simulink model "chap04_01_03_mdl"  (R2013b)
settings: Solver=ode45  StartTime=0.0  StopTime=10.0  RelTol=1e-3
settings Model: Creator=Administrator  LastModifiedBy=sunzx.fnst

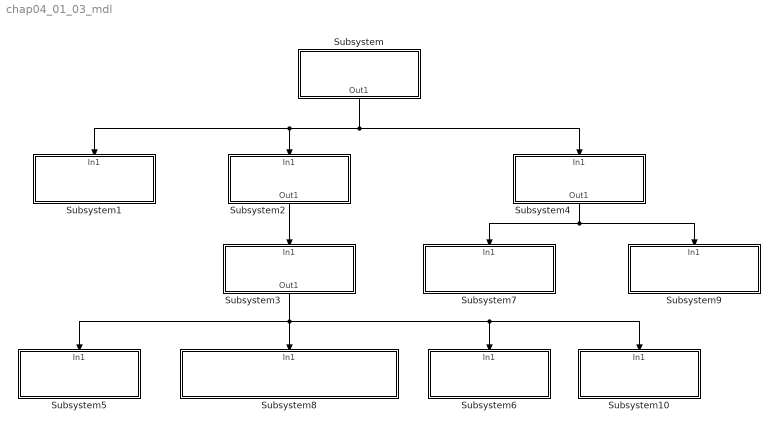
== system chap04_01_03_mdl ==
  Subsystem : Subsystem
      mask Display: disp('Subsystem');
  Subsystem1 : Subsystem
      mask Display: disp('Virtrual Subsystem');
  Subsystem10 : Subsystem
      mask Display: disp('Function-call Subsystem');
  Subsystem2 : Subsystem
      mask Display: disp(['Nonvirtrual Subsystem', char(10), '(Atomic Subsystem)']);
  Subsystem3 : Subsystem
      mask Display: disp('Conditional Subsystem');
  Subsystem4 : Subsystem
      mask Display: disp('Selectable Subsystem');
  Subsystem5 : Subsystem
      mask Display: disp('Triggered Subsystem');
  Subsystem6 : Subsystem
      mask Display: disp('Enable Subsystem');
  Subsystem7 : Subsystem
      mask Display: disp('Configurable Subsystem');
  Subsystem8 : Subsystem
      mask Display: disp('Triggered and Enable Subsystem');
  Subsystem9 : Subsystem
      mask Display: disp('Variant Subsystem');
  wires:
  Subsystem/1(Out1) -> Subsystem1/1(In1), Subsystem2/1(In1), Subsystem4/1(In1)
  Subsystem2/1(Out1) -> Subsystem3/1(In1)
  Subsystem3/1(Out1) -> Subsystem10/1(In1), Subsystem6/1(In1), Subsystem8/1(In1), Subsystem5/1(In1)
  Subsystem4/1(Out1) -> Subsystem9/1(In1), Subsystem7/1(In1)

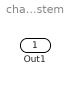
== system chap04_01_03_mdl/Subsystem ==
  Out1 : Outport

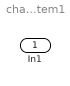
== system chap04_01_03_mdl/Subsystem1 ==
  In1 : Inport

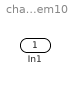
== system chap04_01_03_mdl/Subsystem10 ==
  In1 : Inport

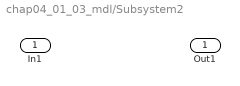
== system chap04_01_03_mdl/Subsystem2 ==
  In1 : Inport
  Out1 : Outport

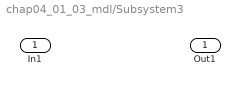
== system chap04_01_03_mdl/Subsystem3 ==
  In1 : Inport
  Out1 : Outport

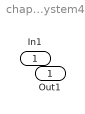
== system chap04_01_03_mdl/Subsystem4 ==
  In1 : Inport
  Out1 : Outport

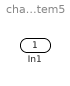
== system chap04_01_03_mdl/Subsystem5 ==
  In1 : Inport

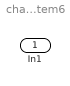
== system chap04_01_03_mdl/Subsystem6 ==
  In1 : Inport

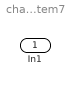
== system chap04_01_03_mdl/Subsystem7 ==
  In1 : Inport

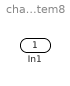
== system chap04_01_03_mdl/Subsystem8 ==
  In1 : Inport

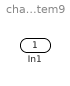
== system chap04_01_03_mdl/Subsystem9 ==
  In1 : Inport
